simulink library "THAMO_6x2"  (R2018a)
settings: Solver=VariableStepAuto  StartTime=0.0  StopTime=10.0  RelTol=1e-3
undefined symbols (not defined in the file): BM, DiameterLastPiece, DPConstant, DPLinear, DPQuadratic, GeodeticHeight, ID, magnitude, MassFlow, Pressure, Temperature, Water
libraries: carnot x11, simulink x10, $bdroot x3
(part 1 of 3)
settings Model: Creator=volkmer  LastModifiedBy=volkmer
settings CodeAppCC: StateflowObjectComments=on

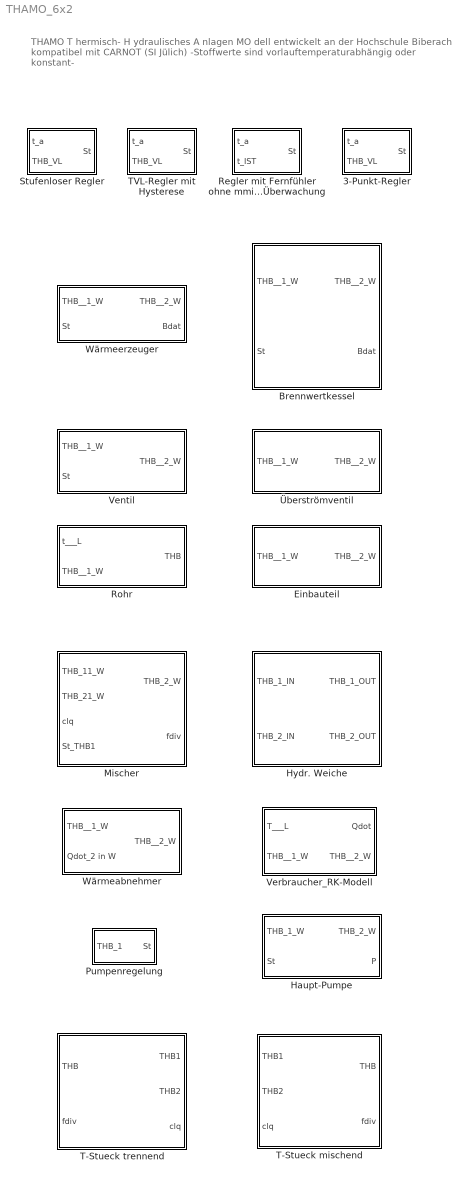
== system THAMO_6x2 ==
  note: THAMO
      | T hermisch- H ydraulisches A nlagen MO dell
      | entwickelt an der Hochschule Biberach
      | kompatibel mit CARNOT (SI Jülich)
      | -Stoffwerte sind vorlauftemperaturabhängig oder konstant-
  3-Punkt-Regler : Subsystem  mask{TVLmax=90, T_HG=50, TVLmin=0, q_S1=40, hyst_S1=6, mmin=3000/30/4.19, tmin=15}
      mask prompts: TVLmax "Vorlauftemperatur bei -16°C"; T_HG "Heizgrenztemperatur"; TVLmin "Vorlauftemperatur bei HG"; q_S1 "Rel. Leistung Stufe 1 in %"; hyst_S1 "Einschaltdifferenz Stufe 1 in K"; mmin "Mindestmassenstrom in kg/s"; tmin "Mindestlaufzeit in min"
      mask DialogControl Container5 Prompt: Heizkurve
      mask DialogControl ParameterGroupVar Prompt: Zusätzliche Parameter
  Brennwertkessel : Subsystem  mask(Condensing Boiler){FUEL=Erdgas, pt_N=20000, V=0.2, Uw=50, AWThw=5, AWTbw=5, P_rel=[20 120], pt_rel=[0.25 1], Lz=1.3, WG_WEhw=4.5, t_hw_A=195, Tamb=20, UV=10, DVB=mit zeta-Wert, kvs=40, zeta=2.5, d=40, m_N=19.44, dp_N=2000}
      mask prompts: FUEL "Brennstoff"; pt_N "Nennleistung in W"; V "Kesselvolumen in m³"; Uw "Wärmedurchgangskoeffizient WÜ in W/m²K"; AWThw "Fläche Kessel-WÜ in m²"; AWTbw "Fläche BW-WÜ in m²"; P_rel "Elektrische Leistung in W (Vektor, index from relative power)"; pt_rel "Rel. Heizleistung in 0..1 (Vektor für P_rel)"; Lz "Luftzahl [-]"; WG_WEhw "Abgasverlust bei t_hw_A in %"; t_hw_A "Abgastemperatur t_hw_A in °C"; Tamb "Umgebungstemperatur in °C"; UV "Wärmeverluste an Umgebung in W/K"; DVB "Druckverlustberechnung"; kvs "kvs-Wert"; zeta "zeta-Wert"; d "Durchmesser in mm"; m_N "Nennmassenstrom in kg/s"; dp_N "Nenndruckverlust in Pa"
      mask help: Multinode one-dimensional model of a boiler. Condensing effects are taken in account by an efficiency lookup table.
      mask Help: web(fullfile(path_carnot('help'),'Condensing_Boiler.html'),'-helpbrowser')
      mask TypeOptions FUEL: Erdgas | Holz (mittel) | Heizoel EL
      mask Callback FUEL:
      | FUEL=1;
      | FUEL=2;
      | FUEL=3;
      mask TypeOptions DVB: mit kvs-Wert | mit zeta-Wert | mit Betriebspunkt
      mask Callback DVB:
      | Auswahl = get_param(gcb,'DVB');
      | Feld = Simulink.Mask.get(gcb);
      | if strcmp(Auswahl,'mit kvs-Wert')
      |     Feld.Parameters(15).Visible = 'on';
      |     Feld.Parameters(16).Visible = 'off';
      |     Feld.Parameters(17).Visible = 'off';
      |     Feld.Parameters(18).Visible = 'off';
      |     Feld.Parameters(19).Visible = 'off';
      |     BM = 1;
      | elseif strcmp(Auswahl,'mit zeta-Wert')
      |     Feld.Parameters(15).Visible = 'off';
      |     Feld.Parameters(16).Visible = 'on';
      |     Feld.Parameters(17).Visible = 'on';
      |     Feld.Parameters(18).Visible = 'off';
      |     Feld.Parameters(19).Visible = 'off';
      |     BM = 2;
      | else
      |     Feld.Parameters(15).Visible = 'off';
      |     Feld.Parameters(16).Visible = 'off';
      |     Feld.Parameters(17).Visible = 'off';
      |     Feld.Parameters(18).Visible = 'on';
      |     Feld.Parameters(19).Visible = 'on';
      |     BM = 3;
      | end
      mask DialogControl DescGroupVar Prompt: Brennwertkessel
      mask DialogControl DescTextVar Prompt: Wärmeerzeuger mit Brennwert-WT für unterschiedliche Brennstoffe
      mask DialogControl ParameterTabVar0 Prompt: Thermisch
      mask DialogControl ParameterTabVar01 Prompt: Effizienz
      mask DialogControl ParameterTabVar012 Prompt: Hydraulisch
      mask Display:
      | plot(-30,0,120,120,[10,90,90,10,10]*0.8,[10,10,20,20,10]*0.8,[80,80,20,20]*0.8,[20,90,90,20]*0.8,[20,70,70,20]*0.8,[24,24,30,30]*0.8,[32,30,28]*0.8,[30,40,30]*0.8,[43,40,38]*0.8,[30,40,30]*0.8,[53,50,47]*0.8,[30,40,30]*0.8,[63,60,57]*0.8,[30,40,30]*0.8,[35,32,30,29,31,36,39,40,37,35]*0.8,[75,69,65,58,50,49,53,59,68,75]*0.8,[57,54,51,51,53,58,62,62,59,57]*0.8,[76,71,67,58,49,48,54,60,69,76]*0.8)
      | port_label('input',1,'THB_1_W')
      | port_label('input',2,'St')
      | port_label('output',1,'THB_2_W')
      | port_label('output',2,'Bdat')
  Einbauteil : Subsystem  mask(Einbauteil){DVB=mit kvs-Wert, kvs=4, zeta=2.5, d=20, m_N=1, dp_N=10^5}
      mask prompts: DVB "Druckverlustberechnung"; kvs "kvs-Wert"; zeta "zeta-Wert"; d "Durchmesser in mm"; m_N "Nennmassenstrom in kg/s"; dp_N "Nenndruckverlust in Pa"
      mask Help: web(fullfile(path_carnot('help'),'Pipe.html'),'-helpbrowser')
      mask TypeOptions DVB: mit kvs-Wert | mit zeta-Wert | mit Betriebspunkt
      mask Callback DVB:
      | Auswahl = get_param(gcb,'DVB');
      | Feld = Simulink.Mask.get(gcb);
      | if strcmp(Auswahl,'mit kvs-Wert')
      |     Feld.Parameters(2).Visible = 'on';
      |     Feld.Parameters(3).Visible = 'off';
      |     Feld.Parameters(4).Visible = 'off';
      |     Feld.Parameters(5).Visible = 'off';
      |     Feld.Parameters(6).Visible = 'off';
      |     BM = 1;
      | elseif strcmp(Auswahl,'mit zeta-Wert')
      |     Feld.Parameters(2).Visible = 'off';
      |     Feld.Parameters(3).Visible = 'on';
      |     Feld.Parameters(4).Visible = 'on';
      |     Feld.Parameters(5).Visible = 'off';
      |     Feld.Parameters(6).Visible = 'off';
      |     BM = 2;
      | else
      |     Feld.Parameters(2).Visible = 'off';
      |     Feld.Parameters(3).Visible = 'off';
      |     Feld.Parameters(4).Visible = 'off';
      |     Feld.Parameters(5).Visible = 'on';
      |     Feld.Parameters(6).Visible = 'on';
      |     BM = 3;
      | end
      mask DialogControl ParameterTabVar0 Prompt: Hydraulik
  Haupt-Pumpe : Subsystem  mask(main pump){a0=651810, a1=5734.30, a2=-346.61, d=0.05, eta_max=80, a=0, mcp=500, p0=4*10^5, IDchk=off, fluid_id=Water, mix=0}
      mask prompts: a0 "Konstanter Kennlinienkoeffizient a0 [Pa]"; a1 "Linearer Kennlinienkoeffizient a1 [Pa*s/kg]"; a2 "Quadratischer Kennlinienkoeffizient a2 [Pa*(s/kg)²]"; d "Anschlussdurchmesser [m]"; eta_max "Max. Wirkungsgrad in %"; a "Wirkungsgradexponent"; mcp "Wärmekapazität in J/K"; p0 "Anlagendruck in Pa"; IDchk "Statischen Druck im System berücksichtigen?"; fluid_id "Fluid"; mix "Mischverhältnis Fluid [0..1]"
      mask help:
      | This is the main pump in a circuit. Every circuit must have exactly ONE 'Pump_Main'. Use the 'pump_additional' blocks if you want to use more pumps.
      | Calculate massflow by solving the equations:
      |     pressure_drop = c + l*mdot + q*(mdot)²
      |     pump_pressure = a0 + a1*mdot +a2*(mdot)²
      |     with: pressure_drop = pump_pressure
      | The system pressure specified as parameter is the pressure at the outlet of the pump. All pressure drops in the circuit will reduce this pressure.
      mask init:
      | ID = IDchk*10000+10001;
      mask Help: web(fullfile(path_carnot('help'),'Pump_Main.html'),'-helpbrowser')
      mask TypeOptions fluid_id: Water | Air | Cotton Oil | Silicone Oil | Water-Glycol Mix | Tyfocor LS | Water (Constant 20°C) | Air (dry+ constant 20°C)
      mask DialogControl ParameterTabVar0 Prompt: Hydraulik
      mask DialogControl Container7 Prompt: Thermisch
      mask DialogControl ParameterTabVar01 Prompt: System
      mask Display:
      | plot(-20,0,100,100,[40,70,40,30,30,40,60,70,70,60,40]*0.8,[70,50,30,40,60,70,70,60,40,30,30]*0.8)
      | 
      | port_label('input',1,'THB_1_W')
      | port_label('input',2,'St')
      | port_label('output',1,'THB_2_W')
      | port_label('output',2,'P')
  Hydr. Weiche : Subsystem  mask{m_HW=500}
      mask prompts: m_HW "Wasserinhalt in kg"
  Mischer : Subsystem  mask{ART=linear, kvs1=4, kvs2=4, dt_V=180}
      mask prompts: ART "Ventilcharakteristik"; kvs1 "kvs THB1-THBg"; kvs2 "kvs THB2-THBg"; dt_V "Mischerlaufzeit in s"
      mask TypeOptions ART: linear | gleichprozentig
      mask Callback ART:
      | ART=1;
      | ART=2;
      mask Display: plot(-25,-5,95,65,[20 45 20 20],[20 30 40 20],[45 70 70 45],[30 20 40 30],[45 35 55 45],[30 10 10 30])
  Pumpenregelung : Subsystem  mask{PUMP=konstantdruckgeregelt, a0=40000, a1=-737, a2=-52000, Vp=20000, Vm=0, nmin=20}
      mask prompts: PUMP "Pumpenbetriebsart"; a0 "constant coefficient in Pa"; a1 "linear coefficient in Pa/(kg/s)"; a2 "quadratic coefficient in Pa/(kg/s)²"; Vp "Vorgabe Förderhöhe (Fußpunkt) in Pa"; Vm "Mindestmassenstrom in kg/s"; nmin "Minimale Drehzahl in %"
      mask TypeOptions PUMP: ungeregelt | konstantdruckgeregelt | proportionaldruckgeregelt
      mask Callback PUMP:
      | PUMP=1;
      | PUMP=2;
      | PUMP=3;
      mask DialogControl DescGroupVar Prompt: Pumpenregelung
      mask DialogControl DescTextVar Prompt: Regelung für eine drehzahlvariable Pumpe
      mask DialogControl ParameterGroupVar Prompt: Reglerdaten
  Regler mit Fernfühler ohne mmin-Überwachung : Subsystem  mask{TVLmax=90, T_HG=50, TVLmin=0, hyst_min=6, tmin=15}
      mask prompts: TVLmax "Vorlauftemperatur bei -16°C"; T_HG "Heizgrenztemperatur"; TVLmin "Vorlauftemperatur bei HG"; hyst_min "Einschaltdifferenz unter Minimalleistung in K"; tmin "Mindestlaufzeit in min"
      mask DialogControl Container5 Prompt: Heizkurve
      mask DialogControl ParameterGroupVar Prompt: Zusätzliche Parameter
  Rohr : Subsystem  mask(Rohr){d=25, L=10, H=0, k=0.03, zeta=0, Uw=20}
      mask prompts: d "Durchmesser in mm"; L "Rohrlänge in m"; H "Wirksame Höhendifferenz in m (offene Systeme)"; k "Rohrrauigkeit in mm"; zeta "zeta-Wert Rohrbögen"; Uw "Wärmeverlust pro m in W/(m*K)"
      mask Help: web(fullfile(path_carnot('help'),'Pipe_Geometry.html'),'-helpbrowser')
      mask DialogControl ParameterTabVar0 Prompt: Hydraulik
      mask DialogControl ParameterTabVar01 Prompt: Thermisch
      mask Display: plot(0,0,90,100,[8,12,16,16,12,8,8],[46,38,46,55,62,55,46],[12,33,48,52,70,73,73,70,50,35,30,12],[38,49,30,30,50,55,65,70,50,70,70,62])
  Stufenloser Regler : Subsystem  mask{TVLmax=90, T_HG=50, TVLmin=0, Kp=50, Ki=6, Kd=3000/30/4.19, q_min=50, hyst_min=6, mmin=3000/30/4.19, tmin=15}
      mask prompts: TVLmax "Vorlauftemperatur bei -16°C"; T_HG "Heizgrenztemperatur"; TVLmin "Vorlauftemperatur bei HG"; Kp "Proportionalbeiwert Kp"; Ki "Integralbeiwert Ki"; Kd "Differentialbeiwert Kd"; q_min "Minimale Leistung in %"; hyst_min "Einschaltdifferenz unter Minimalleistung in K"; mmin "Mindestmassenstrom in kg/s"; tmin "Mindestlaufzeit in min"
      mask DialogControl Container5 Prompt: Heizkurve
      mask DialogControl ParameterGroupVar_copy Prompt: Reglerparameter
      mask DialogControl ParameterGroupVar Prompt: Zusätzliche Parameter
  T-Stueck mischend : Subsystem
      mask Display: plot(-25,-5,95,65,[20 45 20 20],[20 30 40 20],[45 70 70 45],[30 20 40 30],[45 35 55 45],[30 10 10 30])
  T-Stueck trennend : Subsystem  mask(flow diverter, fixed rate){}
      mask help:
      | The block diverts an incoming massflow according to:
      | mdot1 = mdot * fdiv
      | mdot2 = mdot * (1-fdiv)
      | fdiv is limited to the range [0..1]
      mask Help: web(fullfile(path_carnot('help'),'Flow_Diverter.html'),'-helpbrowser')
      mask Display: plot(0,-5,120,65,[20 45 20 20],[20 30 40 20],[45 70 70 45],[30 20 40 30],[45 35 55 45],[30 10 10 30])
  TVL-Regler mit Hysterese : Subsystem  mask{TVLmax=90, T_HG=50, TVLmin=0, hyst_min=6, mmin=3000/30/4.19, tmin=15}
      mask prompts: TVLmax "Vorlauftemperatur bei -16°C"; T_HG "Heizgrenztemperatur"; TVLmin "Vorlauftemperatur bei HG"; hyst_min "Einschaltdifferenz unter Minimalleistung in K"; mmin "Mindestmassenstrom in kg/s"; tmin "Mindestlaufzeit in min"
      mask DialogControl Container5 Prompt: Heizkurve
      mask DialogControl ParameterGroupVar Prompt: Zusätzliche Parameter
  Ventil : Subsystem  mask(Ventil){ART=linear, kvs=5, n_0=0.001, dt_V=180}
      mask prompts: ART "Ventilcharakteristik"; kvs "kvs-Wert in m³/h"; n_0 "Rel. Durchflusskoeffizient"; dt_V "Ventillaufzeit in s"
      mask Help: web(fullfile(path_carnot('help'),'Valve.html'),'-helpbrowser')
      mask TypeOptions ART: linear | gleichprozentig
      mask Callback ART:
      | ART=1;
      | ART=2;
      mask Display: plot(0,10,120,180,[30,70,70,30,30]*0.8,[60,40,60,40,60]*0.8,[60,40]*0.8,[80,80]*0.8,[50,50]*0.8,[50,80]*0.8)
  Verbraucher_RK-Modell : Subsystem  mask(Raumheizeinrichtung){Qdot_N=3*10^6, t_1N=90, t_2N=50, n=1.3, M=500, DVB=mit zeta-Wert, kvs=4, zeta=3, d=150, m_N=1, dp_N=10^5}
      mask prompts: Qdot_N "Nennleistung in W"; t_1N "Nenn-Vorlauftemperatur in °C"; t_2N "Nenn-Rücklauftemperatur in °C"; n "Heizkörperexponent"; M "Wasserinhalt in kg"; DVB "Druckverlustberechnung"; kvs "kvs-Wert"; zeta "zeta-Wert"; d "Durchmesser in mm"; m_N "Nennmassenstrom in kg/s"; dp_N "Nenndruckverlust in Pa"
      mask help: ohne Leistungsvorgabe
      mask Help: web(['file:///' fullfile(path_carnot('help'),'Radiator.html')],'-helpbrowser')
      mask TypeOptions DVB: mit kvs-Wert | mit zeta-Wert | mit Betriebspunkt
      mask Callback DVB:
      | Auswahl = get_param(gcb,'DVB');
      | Feld = Simulink.Mask.get(gcb);
      | if strcmp(Auswahl,'mit kvs-Wert')
      |     Feld.Parameters(7).Visible = 'on';
      |     Feld.Parameters(8).Visible = 'off';
      |     Feld.Parameters(9).Visible = 'off';
      |     Feld.Parameters(10).Visible = 'off';
      |     Feld.Parameters(11).Visible = 'off';
      |     BM = 1;
      | elseif strcmp(Auswahl,'mit zeta-Wert')
      |     Feld.Parameters(7).Visible = 'off';
      |     Feld.Parameters(8).Visible = 'on';
      |     Feld.Parameters(9).Visible = 'on';
      |     Feld.Parameters(10).Visible = 'off';
      |     Feld.Parameters(11).Visible = 'off';
      |     BM = 2;
      | else
      |     Feld.Parameters(7).Visible = 'off';
      |     Feld.Parameters(8).Visible = 'off';
      |     Feld.Parameters(9).Visible = 'off';
      |     Feld.Parameters(10).Visible = 'on';
      |     Feld.Parameters(11).Visible = 'on';
      |     BM = 3;
      | end
      mask DialogControl ParameterTabVar0 Prompt: Thermisch
      mask DialogControl ParameterTabVar01 Prompt: Hydraulik
      mask Display:
      | plot(-20,0,120,90,[20 90 90 20 20],[20 20 70 70 20],[30 30],[25 65],[40 40],[25 65],[50 50],[25 65],[60 60],[25 65],[70 70],[25 65],[80 80],[25 65],[15 20],[25 25],[15 20],[65 65])
      | port_label('input',1,'Troom')
      | port_label('input',2,'THB')
      | port_label('output',1,'Qdot')
      | port_label('output',2,'THB')
  Wärmeabnehmer : Subsystem  mask(Raumheizeinrichtung){M=5, DVB=mit kvs-Wert, kvs=4, zeta=2.5, d=20, m_N=1, dp_N=10^5}
      mask prompts: M "Wasserinhalt in kg"; DVB "Druckverlustberechnung"; kvs "kvs-Wert"; zeta "zeta-Wert"; d "Durchmesser in mm"; m_N "Nennmassenstrom in kg/s"; dp_N "Nenndruckverlust in Pa"
      mask help: mit Leistungsvorgabe (bei Kälte negativ)
      mask Help: web(['file:///' fullfile(path_carnot('help'),'Radiator.html')],'-helpbrowser')
      mask TypeOptions DVB: mit kvs-Wert | mit zeta-Wert | mit Betriebspunkt
      mask Callback DVB:
      | Auswahl = get_param(gcb,'DVB');
      | Feld = Simulink.Mask.get(gcb);
      | if strcmp(Auswahl,'mit kvs-Wert')
      |     Feld.Parameters(3).Visible = 'on';
      |     Feld.Parameters(4).Visible = 'off';
      |     Feld.Parameters(5).Visible = 'off';
      |     Feld.Parameters(6).Visible = 'off';
      |     Feld.Parameters(7).Visible = 'off';
      |     BM = 1;
      | elseif strcmp(Auswahl,'mit zeta-Wert')
      |     Feld.Parameters(3).Visible = 'off';
      |     Feld.Parameters(4).Visible = 'on';
      |     Feld.Parameters(5).Visible = 'on';
      |     Feld.Parameters(6).Visible = 'off';
      |     Feld.Parameters(7).Visible = 'off';
      |     BM = 2;
      | else
      |     Feld.Parameters(3).Visible = 'off';
      |     Feld.Parameters(4).Visible = 'off';
      |     Feld.Parameters(5).Visible = 'off';
      |     Feld.Parameters(6).Visible = 'on';
      |     Feld.Parameters(7).Visible = 'on';
      |     BM = 3;
      | end
      mask DialogControl ParameterTabVar0 Prompt: Thermisch
      mask DialogControl ParameterTabVar01 Prompt: Hydraulik
      mask Display:
      | plot(-20,0,120,90,[20 90 90 20 20],[20 20 70 70 20],[30 30],[25 65],[40 40],[25 65],[50 50],[25 65],[60 60],[25 65],[70 70],[25 65],[80 80],[25 65],[15 20],[25 25],[15 20],[65 65])
      | port_label('input',1,'THB')
      | port_label('input',2,'Qdot_2')
      | port_label('output',1,'THB')
  Wärmeerzeuger : Subsystem  mask(Condensing Boiler){pt_N=20, V=200, FUEL=Erdgas, UV=10, Tamb=20, G=[5 10], t_hw_A=195, WG_WEhw=4.5, Lz=1.3, DVB=mit Betriebspunkt, kvs=40, zeta=2.5, d=40, m_N=1, dp_N=10^5}
      mask prompts: pt_N "Nennleistung in kW"; V "Kesselvolumen in L"; FUEL "Brennstoff"; UV "Wärmeverlust in W/K"; Tamb "Umgebungstemperatur in °C"; G "Grädigkeit Abgas-TRL in K bei Q=[50% 100%]"; t_hw_A "Abgastemperatur t_hw_A in °C"; WG_WEhw "Abgasverlust (ohne Brennwertnutzung) bei Abgastemperatur t_hw_A in %"; Lz "Luftzahl"; DVB "Druckverlustberechnung"; kvs "kvs-Wert"; zeta "zeta-Wert"; d "Durchmesser in mm"; m_N "Nennmassenstrom in kg/s"; dp_N "Nenndruckverlust in Pa"
      mask help: Multinode one-dimensional model of a boiler. Condensing effects are taken in account by an efficiency lookup table.
      mask Help: web(fullfile(path_carnot('help'),'Condensing_Boiler.html'),'-helpbrowser')
      mask TypeOptions FUEL: Erdgas | Holz (mittel) | Heizoel EL
      mask Callback FUEL:
      | FUEL=1;
      | FUEL=2;
      | FUEL=3;
      mask TypeOptions DVB: mit kvs-Wert | mit zeta-Wert | mit Betriebspunkt
      mask Callback DVB:
      | Auswahl = get_param(gcb,'DVB');
      | Feld = Simulink.Mask.get(gcb);
      | if strcmp(Auswahl,'mit kvs-Wert')
      |     Feld.Parameters(11).Visible = 'on';
      |     Feld.Parameters(12).Visible = 'off';
      |     Feld.Parameters(13).Visible = 'off';
      |     Feld.Parameters(14).Visible = 'off';
      |     Feld.Parameters(15).Visible = 'off';
      |     BM = 1;
      | elseif strcmp(Auswahl,'mit zeta-Wert')
      |     Feld.Parameters(11).Visible = 'off';
      |     Feld.Parameters(12).Visible = 'on';
      |     Feld.Parameters(13).Visible = 'on';
      |     Feld.Parameters(14).Visible = 'off';
      |     Feld.Parameters(15).Visible = 'off';
      |     BM = 2;
      | else
      |     Feld.Parameters(11).Visible = 'off';
      |     Feld.Parameters(12).Visible = 'off';
      |     Feld.Parameters(13).Visible = 'off';
      |     Feld.Parameters(14).Visible = 'on';
      |     Feld.Parameters(15).Visible = 'on';
      |     BM = 3;
      | end
      mask DialogControl DescGroupVar Prompt: Brennwertkessel
      mask DialogControl DescTextVar Prompt: Wärmeerzeuger mit Brennwert-WT für unterschiedliche Brennstoffe
      mask DialogControl ParameterTabVar0 Prompt: Thermisch
      mask DialogControl Container10 Prompt: Effizienz
      mask DialogControl ParameterTabVar012 Prompt: Hydraulisch
  Überströmventil : Subsystem  mask(Überströmventil){p0=27111, p1=1330, p2=1889}
      mask prompts: p0 "Durchbrechdruck in Pa"; p1 "Linearer Druckverlustkoeffizient in Pa/(kg/s)"; p2 "Quadratischer Druckverlustkoeffizient in Pa/(kg/s)^2"
      mask Help: web(fullfile(path_carnot('help'),'Valve.html'),'-helpbrowser')

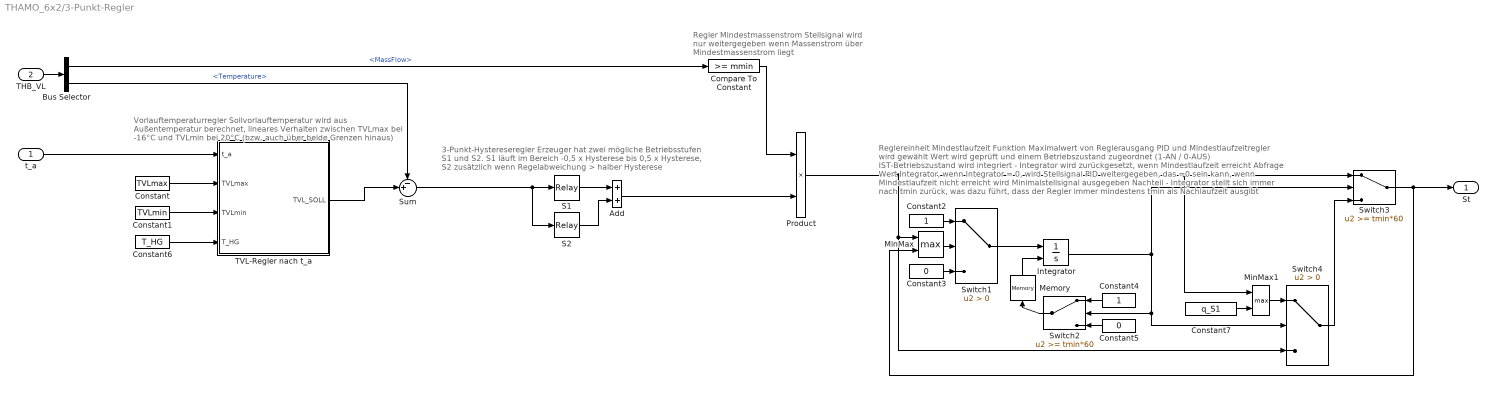
== system THAMO_6x2/3-Punkt-Regler ==
  note: 3-Punkt-Hystereseregler
      |
      | Erzeuger hat zwei mögliche Betriebsstufen
      | S1 und S2. S1 läuft im Bereich -0,5 x Hysterese bis 0,5 x Hysterese, S2 zusätzlich wenn Regelabweichung > halber Hysterese
  note: Vorlauftemperaturregler
      |
      | Sollvorlauftemperatur wird aus Außentemperatur berechnet, lineares Verhalten zwischen TVLmax bei -16°C und TVLmin bei 20°C (bzw. auch über beide Grenzen hinaus)
  note: Regler Mindestmassenstrom
      |
      | Stellsignal wird nur weitergegeben wenn Massenstrom über Mindestmassenstrom liegt
  note: Reglereinheit Mindestlaufzeit
      |
      | Funktion
      | Maximalwert von Reglerausgang PID und Mindestlaufzeitregler wird gewählt
      | Wert wird geprüft und einem Betriebszustand zugeordnet (1-AN / 0-AUS)
      | IST-Betriebszustand wird integriert - Integrator wird zurückgesetzt, wenn Mindestlaufzeit erreicht
      | Abfrage Wert Integrator, wenn Integrator = 0, wird Stellsignal PID weitergegeben, das =0 sein kann, wenn Mindestlaufzeit nicht erreicht wird Minimalstellsignal ausgegeben
      |
      | Nachteil
      | - Integrator stellt sich immer nach tmin zurück, was dazu führt, dass der Regler immer mindestens tmin als Nachlaufzeit ausgibt
  t_a : Inport
  THB_VL : Inport  Port=2
  Add : Sum
  Bus Selector : BusSelector  OutputSignals=MassFlow,Temperature
  Compare To Constant : simulink/Logic and Bit Operations/Compare To Constant  relop=>=  const=mmin  OutDataTypeStr=boolean
  Constant : Constant  Value=TVLmax
  Constant1 : Constant  Value=TVLmin
  Constant2 : Constant
  Constant3 : Constant  Value=0
  Constant4 : Constant
  Constant5 : Constant  Value=0
  Constant6 : Constant  Value=T_HG
  Constant7 : Constant  Value=q_S1
  Integrator : Integrator  ExternalReset=level hold
  Memory : Memory  InitialCondition=1
  MinMax : MinMax  Function=max  Inputs=2
  MinMax1 : MinMax  Function=max  Inputs=2
  Product : Product
  S1 : Relay  OnSwitchValue=hyst_S1*0.5  OffSwitchValue=-hyst_S1*0.5  OnOutputValue=q_S1/100
  S2 : Relay  OnSwitchValue=hyst_S1  OffSwitchValue=-hyst_S1*0.5  OnOutputValue=1-q_S1/100
  Sum : Sum  Inputs=-+|
  Switch1 : Switch  Criteria=u2 > Threshold
  Switch2 : Switch  Threshold=tmin*60
  Switch3 : Switch  Threshold=tmin*60
  Switch4 : Switch  Criteria=u2 > Threshold
  TVL-Regler nach t_a : MATLAB Function  TreatAsAtomicUnit=on
  St : Outport
  wires:
  Memory/1 -> Integrator/2
  TVL-Regler nach t_a/1(TVL_SOLL) -> Sum/2
  Compare To Constant/1 -> Product/1
  Bus Selector/1 -> Compare To Constant/1  "<MassFlow>"
  Product/1 -> MinMax1/1, Switch3/1, Switch4/3, MinMax/1
  Constant1/1 -> TVL-Regler nach t_a/3(TVLmin)
  Constant/1 -> TVL-Regler nach t_a/2(TVLmax)
  t_a/1 -> TVL-Regler nach t_a/1(t_a)
  Bus Selector/2 -> Sum/1  "<Temperature>"
  THB_VL/1 -> Bus Selector/1
  Constant2/1 -> Switch1/1
  Constant3/1 -> Switch1/3
  Switch1/1 -> Integrator/1
  Switch2/1 -> Memory/1
  Constant4/1 -> Switch2/1
  Constant5/1 -> Switch2/3
  Integrator/1 -> Switch2/2, Switch4/2, Switch3/2
  Switch3/1 -> St/1, MinMax/2
  Switch4/1 -> Switch3/3
  MinMax/1 -> Switch1/2
  MinMax1/1 -> Switch4/1
  Constant7/1 -> MinMax1/2
  Add/1 -> Product/2
  S2/1 -> Add/2
  Sum/1 -> S1/1, S2/1
  S1/1 -> Add/1
  Constant6/1 -> TVL-Regler nach t_a/4(T_HG)

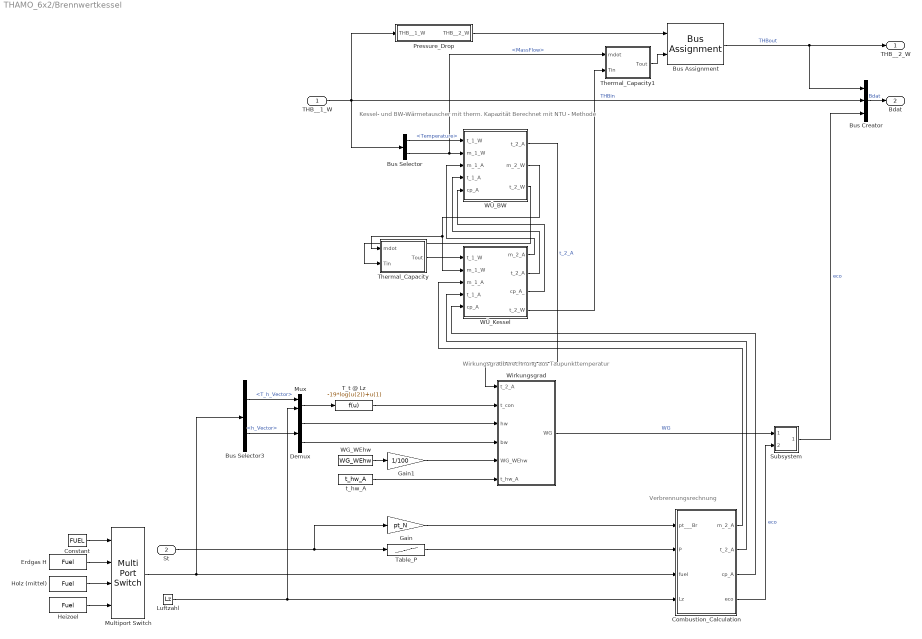
== system THAMO_6x2/Brennwertkessel ==
  note: Wirkungsgradberechnung aus Taupunkttemperatur
  note: Verbrennungsrechnung
  note: Kessel- und BW-Wärmetauscher mit therm. Kapazität
      |
      | Berechnet mit NTU - Methode
  THB__1_W : Inport
  St : Inport  Port=2
  Bus Assignment : BusAssignment  AssignedSignals=Temperature
  Bus Creator : BusCreator  Inputs=3
  Bus Selector : BusSelector  OutputSignals=Temperature,MassFlow
  Bus Selector3 : BusSelector  OutputSignals=T_h_Vector,h_Vector
  Combustion_Calculation : Subsystem  TreatAsAtomicUnit=on
  Constant : Constant  Value=FUEL
  Demux : Demux  Outputs=2
  Erdgas H : carnot/Source/Energy/Fuel  ft=1  t=20  ls=15.59  p=1e5  h_values=[38.5 43]*10^6  tc=57.53  price=1  mass=[0.22 0.70 0.05 0 0.03 0]
  Gain : Gain  Gain=pt_N
  Gain1 : Gain  Gain=1/100
  Heizoel : carnot/Source/Energy/Fuel  ft=2  t=20  ls=15.94  p=1e5  h_values=[42.6 45.4]*10^6  tc=50.37  price=1  mass=[0.13 0.87 0 0 0 0]
  Holz (mittel) : carnot/Source/Energy/Fuel  ft=3  t=20  ls=6.54  p=1e5  h_values=[15.1 19]*10^6  tc=67.5  price=1  mass=[0.06 0.5 0.44 0 0 0]
  Luftzahl : Constant  Value=Lz
  Multiport Switch : MultiPortSwitch
  Mux : Mux  Inputs=2
  Pressure_Drop : Subsystem  mask(fixed pressure drop){}
      mask help:
      | Constant parameters for pressure drop in a flow.
      | dp = c + l*mdot + q*mdot²
      | Calculation is done for ID > 10000 (dp = f(l, q), c is neglected) and ID > 20000 (dp = f(c,l,q)).
      | Applied directly to the THB bus.
      mask Help: web(fullfile(path_carnot('help'),'Pressure_Drop_Fix.html'),'-helpbrowser')
  Subsystem : Subsystem
  T_t @ Lz : Fcn  Expr=-19*log(u(2))+u(1)
  Table_P : Lookup_n-D  NumberOfTableDimensions=1  BreakpointsForDimension1=[0 pt_rel]  Table=[0 P_rel]  InternalRulePriority=Speed  InputSameDT=on
  Thermal_Capacity : Subsystem  mask(Thermal Capacity){}
      mask help: Basic one node model of a thermal mass using the differential equation:
      mask Help: web(fullfile(path_carnot('help'),'Thermal_Capacity.html'),'-helpbrowser')
  Thermal_Capacity1 : Subsystem  mask(Thermal Capacity){}
      mask help: Basic one node model of a thermal mass using the differential equation:
      mask Help: web(fullfile(path_carnot('help'),'Thermal_Capacity.html'),'-helpbrowser')
  WG_WEhw : Constant  Value=WG_WEhw
  Wirkungsgrad : MATLAB Function  TreatAsAtomicUnit=on
  WÜ_BW : Subsystem
  WÜ_Kessel : Subsystem
  t_hw_A : Constant  Value=t_hw_A
  THB__2_W : Outport
  Bdat : Outport  Port=2
  wires:
  Combustion_Calculation/2(t_2_A) -> WÜ_Kessel/4(t_1_A)
  Constant/1 -> Multiport Switch/1
  Heizoel/1 -> Multiport Switch/4
  Holz (mittel)/1 -> Multiport Switch/3
  Erdgas H/1 -> Multiport Switch/2
  Combustion_Calculation/1(m_2_A) -> WÜ_Kessel/3(m_1_A)
  WÜ_BW/1(t_2_A) -> Wirkungsgrad/1(t_2_A)  "t_2_A"
  Gain1/1 -> Wirkungsgrad/5(WG_WEhw)
  t_hw_A/1 -> Wirkungsgrad/6(t_hw_A)
  WG_WEhw/1 -> Gain1/1
  T_t @ Lz/1 -> Wirkungsgrad/2(t_con)
  Luftzahl/1 -> Mux/2, Combustion_Calculation/4(Lz)
  Mux/1 -> T_t @ Lz/1
  Demux/2 -> Wirkungsgrad/4(bw)
  Demux/1 -> Wirkungsgrad/3(hw)
  Bus Selector3/2 -> Demux/1  "<h_Vector>"
  Bus Selector3/1 -> Mux/1  "<T_h_Vector>"
  Table_P/1 -> Combustion_Calculation/2(P)
  Bus Creator/1 -> Bdat/1  "Bdat"
  THB__1_W/1 -> Bus Selector/1, Pressure_Drop/1(THB__1_W), Bus Creator/2  "THBin"
  Bus Assignment/1 -> THB__2_W/1, Bus Creator/1  "THBout"
  St/1 -> Table_P/1, Gain/1
  Multiport Switch/1 -> Bus Selector3/1, Combustion_Calculation/3(fuel)
  Pressure_Drop/1(THB__2_W) -> Bus Assignment/1
  Gain/1 -> Combustion_Calculation/1(pt___Br)
  Bus Selector/2 -> Thermal_Capacity1/1(mdot), WÜ_BW/2(m_1_W)  "<MassFlow>"
  WÜ_BW/2(m_2_W) -> WÜ_Kessel/2(m_1_W), Thermal_Capacity/1(mdot)
  Combustion_Calculation/3(cp_A) -> WÜ_Kessel/5(cp_A)
  WÜ_Kessel/3(cp_A_) -> WÜ_BW/5(cp_A)
  Wirkungsgrad/1(WG) -> Subsystem/1(WG)  "WG"
  Combustion_Calculation/4(eco) -> Subsystem/2(eco_in)  "eco"
  Subsystem/1(eco) -> Bus Creator/3  "eco"
  WÜ_Kessel/1(m_2_A) -> WÜ_BW/3(m_1_A)
  Bus Selector/1 -> WÜ_BW/1(t_1_W)  "<Temperature>"
  WÜ_Kessel/2(t_2_A) -> WÜ_BW/4(t_1_A)
  WÜ_BW/3(t_2_W) -> Thermal_Capacity/2(Tin)
  WÜ_Kessel/4(t_2_W) -> Thermal_Capacity1/2(Tin)
  Thermal_Capacity/1(Tout) -> WÜ_Kessel/1(t_1_W)
  Thermal_Capacity1/1(Tout) -> Bus Assignment/2

== system THAMO_6x2/Einbauteil ==
  THB__1_W : Inport
  Pressure_Drop : $bdroot/Brennwertkessel/Pressure_Drop
  THB__2_W : Outport
  wires:
  Pressure_Drop/1 -> THB__2_W/1
  THB__1_W/1 -> Pressure_Drop/1

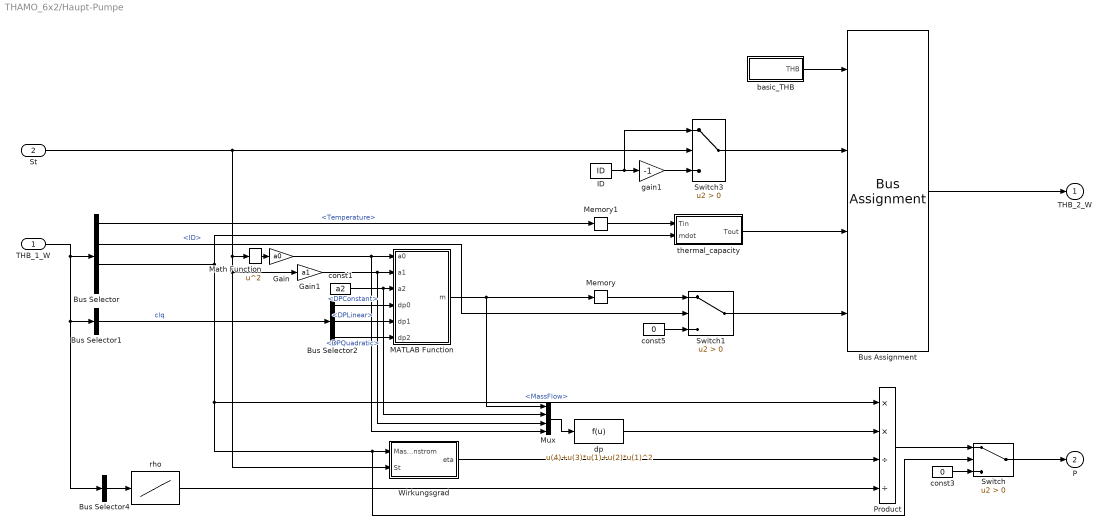
== system THAMO_6x2/Haupt-Pumpe ==
  THB_1_W : Inport
  St : Inport  Port=2
  Bus Assignment : BusAssignment  AssignedSignals=ID,Temperature,MassFlow
  Bus Selector : BusSelector  OutputSignals=Temperature,ID,MassFlow,Pressure
  Bus Selector1 : BusSelector  OutputSignals=DPQuadratic,DPLinear,DPConstant  OutputAsBus=on
  Bus Selector2 : BusSelector  OutputSignals=DPConstant,DPLinear,DPQuadratic
  Bus Selector4 : BusSelector  OutputSignals=Temperature  OutputAsBus=on
  Gain : Gain  Gain=a0
  Gain1 : Gain  Gain=a1
  ID : Constant  Value=ID
  MATLAB Function : MATLAB Function  TreatAsAtomicUnit=on
  Math Function : Math  Operator=square  SaturateOnIntegerOverflow=on
  Memory : Memory  InitialCondition=10^-9
  Memory1 : Memory  InitialCondition=20
  Mux : Mux
  Product : Product  Inputs=**//  SaturateOnIntegerOverflow=on  InputSameDT=on  OutDataTypeStr=Inherit: Same as first input
  Switch : Switch  Criteria=u2 > Threshold
  Switch1 : Switch  Criteria=u2 > Threshold  SaturateOnIntegerOverflow=on  InputSameDT=on
  Switch3 : Switch  Criteria=u2 > Threshold  SaturateOnIntegerOverflow=on  InputSameDT=on
  Wirkungsgrad : Subsystem
  basic_THB : Subsystem  mask(basic THB){t=20, mdot=0, p=p0, ID=Pressure Drop from Massflow, fluid=Water, mix=mix, mix2=0, mix3=0, dia=d, hgt=0}
      mask prompts: t "temperature [°C]"; mdot "massflow [kg/s]"; p "pressure [Pa]"; ID "ID for pressure drop calculation"; mix "fluid mixture [0..1]"; mix2 "fluid mixture 2 [0..1]"; mix3 "fluid mixture 3 [0..1]"; dia "diameter [m]"; hgt "Static height in m"
      mask help:
      | Create a constant Thermo-Hydraulic-Vector.
      | Pressure drop calculation mode (defined by ID):
      |     1 ..  9999 no pressure drop (dp)
      | 10001 .. 19999 dp caused by flowrate
      | 20001 .. inf   dp by flowrate and static height
      mask Help: web(fullfile(path_carnot('help'),'basic_THB.html'),'-helpbrowser')
      mask TypeOptions t: const24/Value
      mask TypeOptions mdot: const25/Value
      mask TypeOptions p: const26/Value
      mask TypeOptions ID: const21/mID
      mask TypeOptions fluid: const27/fluid
      mask TypeOptions mix: const28/Value
      mask TypeOptions mix2: const2/Value
      mask TypeOptions mix3: const3/Value
      mask TypeOptions dia: const29/Value
      mask TypeOptions hgt: const1/Value
      mask DialogControl ParameterTabVar0 Prompt: Hydraulic
      mask DialogControl ParameterTabVar01 Prompt: Fluid
      mask DialogControl ParameterTabVar012 Prompt: Geometry
  const1 : Constant  Value=a2
  const3 : Constant  Value=0
  const5 : Constant  Value=0
  dp : Fcn  Expr=u(4)+u(3)*u(1)+u(2)*u(1)^2
  gain1 : Gain  Gain=-1  SaturateOnIntegerOverflow=on  OutDataTypeStr=Inherit: Same as input  ParamDataTypeStr=Inherit: Same as input
  rho : Lookup_n-D  NumberOfTableDimensions=1  BreakpointsForDimension1=[0,10,20,30,40,50,60,70,80,90,100]  Table=[999.84,999.7,998.2,995.64,992.21,988.03,983.19,977.76,971.79,965.3,958.35]  InternalRulePriority=Speed  RndMeth=Simplest  InputSameDT=on
  thermal_capacity : Subsystem  mask(Thermal Capacity){}
      mask help: Basic one node model of a thermal mass using the differential equation:
      mask Help: web(fullfile(path_carnot('help'),'Thermal_Capacity.html'),'-helpbrowser')
  THB_2_W : Outport
  P : Outport  Port=2
  wires:
  Bus Selector4/1 -> rho/1
  Memory1/1 -> thermal_capacity/1(Tin)
  Gain/1 -> Mux/4, MATLAB Function/1(a0)
  const1/1 -> Mux/2, MATLAB Function/3(a2)
  Bus Selector2/3 -> MATLAB Function/6(dp2)  "<DPQuadratic>"
  Bus Selector2/2 -> MATLAB Function/5(dp1)  "<DPLinear>"
  Bus Selector2/1 -> MATLAB Function/4(dp0)  "<DPConstant>"
  MATLAB Function/1(m) -> Mux/1, Memory/1
  Memory/1 -> Switch1/1
  Gain1/1 -> Mux/3, MATLAB Function/2(a1)
  Math Function/1 -> Gain/1
  Wirkungsgrad/1(eta) -> Product/3
  rho/1 -> Product/4
  Bus Selector/3 -> thermal_capacity/2(mdot), Wirkungsgrad/1(Massenstrom), Switch/2, Product/1  "<MassFlow>"
  Bus Selector1/1 -> Bus Selector2/1  "clq"
  THB_1_W/1 -> Bus Selector4/1, Bus Selector1/1, Bus Selector/1
  Switch1/1 -> Bus Assignment/4
  Switch3/1 -> Bus Assignment/2
  Bus Assignment/1 -> THB_2_W/1
  basic_THB/1(THB) -> Bus Assignment/1
  const5/1 -> Switch1/3
  gain1/1 -> Switch3/3
  ID/1 -> gain1/1, Switch3/1
  St/1 -> Switch3/2, Wirkungsgrad/2(St), Gain1/1, Math Function/1
  Bus Selector/2 -> Switch1/2  "<ID>"
  Product/1 -> Switch/1
  thermal_capacity/1(Tout) -> Bus Assignment/3
  Bus Selector/1 -> Memory1/1  "<Temperature>"
  Switch/1 -> P/1
  const3/1 -> Switch/3
  Mux/1 -> dp/1
  dp/1 -> Product/2

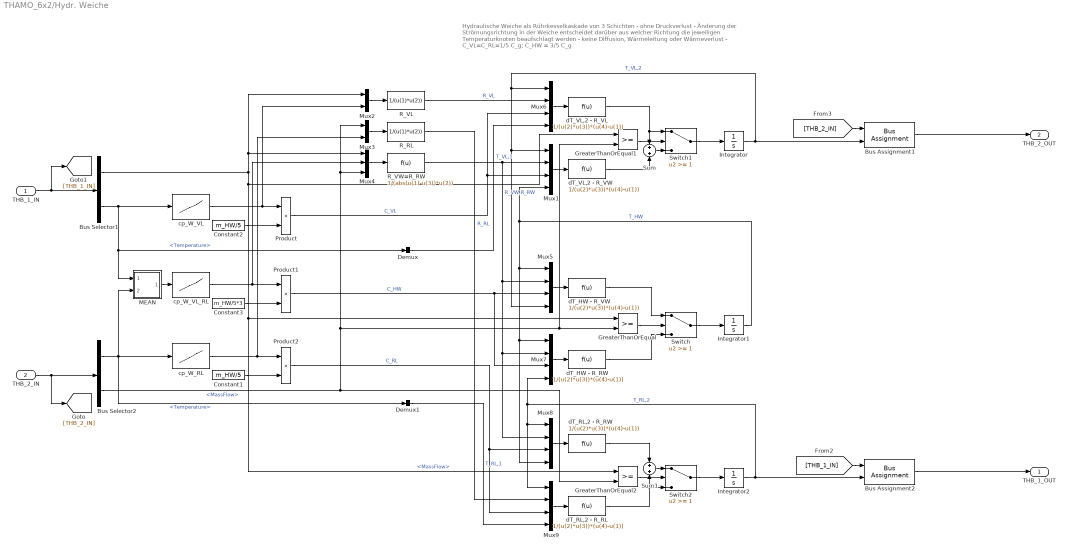
== system THAMO_6x2/Hydr. Weiche ==
  note: Hydraulische Weiche als Rührkesselkaskade von 3 Schichten
      | - ohne Druckverlust
      | - Änderung der Strömungsrichtung in der Weiche entscheidet darüber aus welcher Richtung die jeweiligen Temperaturknoten beaufschlagt werden
      | - keine Diffusion, Wärmeleitung oder Wärmeverlust
      | - C_VL=C_RL=1/5 C_g; C_HW = 3/5 C_g
  THB_1_IN : Inport
  THB_2_IN : Inport  Port=2
  Bus Assignment1 : BusAssignment  AssignedSignals=Temperature
  Bus Assignment2 : BusAssignment  AssignedSignals=Temperature
  Bus Selector1 : BusSelector  OutputSignals=MassFlow,Temperature
  Bus Selector2 : BusSelector  OutputSignals=Temperature,MassFlow
  Constant1 : Constant  Value=m_HW/5
  Constant2 : Constant  Value=m_HW/5
  Constant3 : Constant  Value=m_HW/5*3
  Demux : Demux  Outputs=1
  Demux1 : Demux  Outputs=1
  GreaterThanOrEqual : RelationalOperator  OutDataTypeStr=boolean  RndMeth=Simplest
  GreaterThanOrEqual1 : RelationalOperator  OutDataTypeStr=boolean  RndMeth=Simplest
  GreaterThanOrEqual2 : RelationalOperator  OutDataTypeStr=boolean  RndMeth=Simplest
  Integrator : Integrator  InitialCondition=20
  Integrator1 : Integrator  InitialCondition=20
  Integrator2 : Integrator  InitialCondition=20
  MEAN : Subsystem
  Mux{1,5..9} (6 alike) : Mux
  Mux2 : Mux  Inputs=2
  Mux3 : Mux  Inputs=2
  Mux4 : Mux  Inputs=3
  Product : Product
  Product1 : Product
  Product2 : Product
  R_RL : Fcn  Expr=1/(u(1)*u(2))
  R_VL : Fcn  Expr=1/(u(1)*u(2))
  R_VW=R_RW : Fcn  Expr=1/(abs(u(1)-u(3))*u(2))
  Sum : Sum  Inputs=+|+
  Sum1 : Sum  Inputs=+|+
  Switch : Switch  Threshold=1
  Switch1 : Switch  Threshold=1
  Switch2 : Switch  Threshold=1
  cp_W_RL : Lookup_n-D  NumberOfTableDimensions=1  BreakpointsForDimension1=[0,10,20,30,40,50,60,70,80,90,100]  Table=[4218,4192,4182,4179,4179,4181,4184,4190,4196,4205,4216]  InternalRulePriority=Speed  RndMeth=Simplest  InputSameDT=on
  cp_W_VL : Lookup_n-D  NumberOfTableDimensions=1  BreakpointsForDimension1=[0,10,20,30,40,50,60,70,80,90,100]  Table=[4218,4192,4182,4179,4179,4181,4184,4190,4196,4205,4216]  InternalRulePriority=Speed  RndMeth=Simplest  InputSameDT=on
  cp_W_VL_RL : Lookup_n-D  NumberOfTableDimensions=1  BreakpointsForDimension1=[0,10,20,30,40,50,60,70,80,90,100]  Table=[4218,4192,4182,4179,4179,4181,4184,4190,4196,4205,4216]  InternalRulePriority=Speed  RndMeth=Simplest  InputSameDT=on
  dT_HW - R_RW : Fcn  Expr=1/(u(2)*u(3))*(u(4)-u(1))
  dT_HW - R_VW : Fcn  Expr=1/(u(2)*u(3))*(u(4)-u(1))
  dT_RL,2 - R_RL : Fcn  Expr=1/(u(2)*u(3))*(u(4)-u(1))
  dT_RL,2 - R_RW : Fcn  Expr=1/(u(2)*u(3))*(u(4)-u(1))
  dT_VL,2 - R_VL : Fcn  Expr=1/(u(2)*u(3))*(u(4)-u(1))
  dT_VL,2 - R_VW : Fcn  Expr=1/(u(2)*u(3))*(u(4)-u(1))
  THB_1_OUT : Outport
  THB_2_OUT : Outport  Port=2
  wires:
  Bus Assignment2/1 -> THB_1_OUT/1
  Bus Assignment1/1 -> THB_2_OUT/1
  dT_HW - R_RW/1 -> Switch/3
  dT_HW - R_VW/1 -> Switch/1
  dT_RL,2 - R_RL/1 -> Sum1/2, Switch2/3
  dT_RL,2 - R_RW/1 -> Sum1/1
  Sum1/1 -> Switch2/1
  dT_VL,2 - R_VW/1 -> Sum/2
  dT_VL,2 - R_VL/1 -> Sum/1, Switch1/1
  Sum/1 -> Switch1/3
  Switch2/1 -> Integrator2/1
  Switch1/1 -> Integrator/1
  GreaterThanOrEqual2/1 -> Switch2/2
  GreaterThanOrEqual1/1 -> Switch1/2
  Switch/1 -> Integrator1/1
  GreaterThanOrEqual/1 -> Switch/2
  R_RL/1 -> Mux9/2  "R_RL"
  Integrator2/1 -> Mux7/4, Mux9/1, Mux8/1, Bus Assignment2/2  "T_RL,2"
  Integrator1/1 -> Mux1/4, Mux8/4, Mux7/1, Mux5/1  "T_HW"
  Integrator/1 -> Mux1/1, Mux5/4, Mux6/1, Bus Assignment1/2  "T_VL,2"
  R_VW=R_RW/1 -> Mux1/2, Mux8/2, Mux7/2, Mux5/2  "R_VW,R_RW"
  R_VL/1 -> Mux6/2  "R_VL"
  Mux9/1 -> dT_RL,2 - R_RL/1
  Mux8/1 -> dT_RL,2 - R_RW/1
  Mux7/1 -> dT_HW - R_RW/1
  Mux5/1 -> dT_HW - R_VW/1
  Mux1/1 -> dT_VL,2 - R_VW/1
  Mux6/1 -> dT_VL,2 - R_VL/1
  Product2/1 -> Mux9/3, Mux8/3  "C_RL"
  Product/1 -> Mux1/3, Mux6/3  "C_VL"
  Product1/1 -> Mux5/3, Mux7/3  "C_HW"
  Demux/1 -> Mux6/4  "T_VL,1"
  Demux1/1 -> Mux9/4  "T_RL,1"
  Bus Selector1/1 -> Mux4/1, Mux2/1, GreaterThanOrEqual1/1, GreaterThanOrEqual/1, GreaterThanOrEqual2/1  "<MassFlow>"
  Bus Selector2/2 -> Mux4/3, Mux3/1, GreaterThanOrEqual/2, GreaterThanOrEqual1/2, GreaterThanOrEqual2/2  "<MassFlow>"
  Mux4/1 -> R_VW=R_RW/1
  Mux3/1 -> R_RL/1
  Mux2/1 -> R_VL/1
  [THB_2_IN] -> Bus Assignment1/1
  [THB_1_IN] -> Bus Assignment2/1
  cp_W_RL/1 -> Mux3/2, Product2/1
  Constant1/1 -> Product2/2
  cp_W_VL_RL/1 -> Mux4/2, Product1/1
  Constant3/1 -> Product1/2
  cp_W_VL/1 -> Mux2/2, Product/1
  Constant2/1 -> Product/2
  MEAN/1(Tm) -> cp_W_VL_RL/1
  Bus Selector2/1 -> cp_W_RL/1, Demux1/1, MEAN/2(T_RL)  "<Temperature>"
  Bus Selector1/2 -> cp_W_VL/1, Demux/1, MEAN/1(T_VL)  "<Temperature>"
  THB_1_IN/1 -> Bus Selector1/1, [THB_1_IN]
  THB_2_IN/1 -> Bus Selector2/1, [THB_2_IN]

== system THAMO_6x2/Mischer ==
  note: Zwei Ventile mit möglicherweise unterschiedlichen kvs-Werten (aber gleicher Charakteristik und Laufzeit), wobei St für die Strömung THB_11_W angesetzt wird und das Ventil in THB_21_W entsprechend gegenläufig arbeitet
  THB_11_W : Inport
  THB_21_W : Inport  Port=2
  clq : Inport  Port=3
  St_THB1 : Inport  Port=4
  Constant : Constant
  Sum : Sum  Inputs=-+|
  T-Stueck mischend : $bdroot/T-Stueck mischend  SystemSampleTime=-1
  Ventil : Subsystem  mask(Ventil){kvs=kvs1, n_0=0.01, dt_V=dt_V}
      mask prompts: kvs "kvs-Wert in m³/h"; n_0 "Rel. Durchflusskoeffizient"; dt_V "Ventillaufzeit in s"
      mask Help: web(fullfile(path_carnot('help'),'Valve.html'),'-helpbrowser')
      mask Display: plot(0,10,120,180,[30,70,70,30,30]*0.8,[60,40,60,40,60]*0.8,[60,40]*0.8,[80,80]*0.8,[50,50]*0.8,[50,80]*0.8)
  Ventil1 : Subsystem  mask(Ventil){kvs=kvs2, n_0=0.01, dt_V=dt_V}
      mask prompts: kvs "kvs-Wert in m³/h"; n_0 "Rel. Durchflusskoeffizient"; dt_V "Ventillaufzeit in s"
      mask Help: web(fullfile(path_carnot('help'),'Valve.html'),'-helpbrowser')
      mask Display: plot(0,10,120,180,[30,70,70,30,30]*0.8,[60,40,60,40,60]*0.8,[60,40]*0.8,[80,80]*0.8,[50,50]*0.8,[50,80]*0.8)
  THB_2_W : Outport
  fdiv : Outport  Port=2
  wires:
  THB_21_W/1 -> Ventil1/1(THB__1_W)
  Ventil/1(THB__2_W) -> T-Stueck mischend/1
  Ventil1/1(THB__2_W) -> T-Stueck mischend/2
  THB_11_W/1 -> Ventil/1(THB__1_W)
  T-Stueck mischend/2 -> fdiv/1
  T-Stueck mischend/1 -> THB_2_W/1
  St_THB1/1 -> Sum/1, Ventil/2(St)
  clq/1 -> T-Stueck mischend/3
  Sum/1 -> Ventil1/2(St)
  Constant/1 -> Sum/2

== system THAMO_6x2/Pumpenregelung ==
  THB_1 : Inport
  Bus Selector : BusSelector  OutputSignals=DPConstant,DPLinear,DPQuadratic
  Constant : Constant  Value=a0
  Constant1 : Constant  Value=a1
  Constant2 : Constant  Value=a2
  Constant3 : Constant  Value=Vp
  Constant4 : Constant  Value=Vm
  Constant5 : Constant  Value=PUMP
  Constant6 : Constant  Value=0
  MATLAB Function : MATLAB Function  TreatAsAtomicUnit=on
  Memory : Memory  InitialCondition=1
  Saturation : Saturate  UpperLimit=1  LowerLimit=0  LinearizeAsGain=off
  Switch : Switch  Criteria=u2 > Threshold  Threshold=nmin/100
  St : Outport
  wires:
  MATLAB Function/1(St) -> Switch/1, Switch/2
  Switch/1 -> Saturation/1
  THB_1/1 -> Bus Selector/1
  Bus Selector/1 -> MATLAB Function/1(dp0)  "<DPConstant>"
  Bus Selector/2 -> MATLAB Function/2(dp1)  "<DPLinear>"
  Bus Selector/3 -> MATLAB Function/3(dp2)  "<DPQuadratic>"
  Constant5/1 -> MATLAB Function/4(PUMP)
  Constant/1 -> MATLAB Function/5(a0)
  Constant1/1 -> MATLAB Function/6(a1)
  Constant2/1 -> MATLAB Function/7(a2)
  Constant3/1 -> MATLAB Function/8(Vp)
  Constant4/1 -> MATLAB Function/9(Vm)
  Saturation/1 -> Memory/1
  Memory/1 -> St/1
  Constant6/1 -> Switch/3

== system THAMO_6x2/Regler mit Fernfühler ohne mmin-Überwachung ==
  note: Hystereseregler
      |
      | Erzeuger wird zwischen 0 und 1 mit Hysterese stufig geschalten
  note: Vorlauftemperaturregler
      |
      | Sollvorlauftemperatur wird aus Außentemperatur berechnet, lineares Verhalten zwischen TVLmax bei -16°C und TVLmin bei 20°C (bzw. auch über beide Grenzen hinaus)
  note: Reglereinheit Mindestlaufzeit
      |
      | Funktion
      | Maximalwert von Reglerausgang PID und Mindestlaufzeitregler wird gewählt
      | Wert wird geprüft und einem Betriebszustand zugeordnet (1-AN / 0-AUS)
      | IST-Betriebszustand wird integriert - Integrator wird zurückgesetzt, wenn Mindestlaufzeit erreicht
      | Abfrage Wert Integrator, wenn Integrator = 0, wird Stellsignal PID weitergegeben, das =0 sein kann, wenn Mindestlaufzeit nicht erreicht wird Minimalstellsignal ausgegeben
      |
      | Nachteil
      | - Integrator stellt sich immer nach tmin zurück, was dazu führt, dass der Regler immer mindestens tmin als Nachlaufzeit ausgibt
  t_a : Inport
  t_IST : Inport  Port=2
  Constant : Constant  Value=TVLmax
  Constant1 : Constant  Value=TVLmin
  Constant2 : Constant
  Constant3 : Constant  Value=0
  Constant4 : Constant
  Constant5 : Constant  Value=0
  Constant6 : Constant  Value=T_HG
  Constant7 : Constant
  Integrator : Integrator  ExternalReset=level hold
  Memory : Memory  InitialCondition=1
  MinMax : MinMax  Function=max  Inputs=2
  MinMax1 : MinMax  Function=max  Inputs=2
  Relay : Relay  OnSwitchValue=hyst_min/2  OffSwitchValue=-hyst_min/2
  Sum : Sum  Inputs=-+|
  Switch1 : Switch  Criteria=u2 > Threshold
  Switch2 : Switch  Threshold=tmin*60
  Switch3 : Switch  Threshold=tmin*60
  Switch4 : Switch  Criteria=u2 > Threshold
  TVL-Regler nach t_a : MATLAB Function  TreatAsAtomicUnit=on
  St : Outport
  wires:
  Memory/1 -> Integrator/2
  Sum/1 -> Relay/1
  TVL-Regler nach t_a/1(TVL_SOLL) -> Sum/2
  Relay/1 -> Switch4/3, MinMax/1, MinMax1/1, Switch3/1
  Constant1/1 -> TVL-Regler nach t_a/3(TVLmin)
  Constant/1 -> TVL-Regler nach t_a/2(TVLmax)
  t_a/1 -> TVL-Regler nach t_a/1(t_a)
  t_IST/1 -> Sum/1
  Constant2/1 -> Switch1/1
  Constant3/1 -> Switch1/3
  Switch1/1 -> Integrator/1
  Switch2/1 -> Memory/1
  Constant4/1 -> Switch2/1
  Constant5/1 -> Switch2/3
  Integrator/1 -> Switch2/2, Switch4/2, Switch3/2
  Switch3/1 -> St/1, MinMax/2
  Switch4/1 -> Switch3/3
  MinMax/1 -> Switch1/2
  MinMax1/1 -> Switch4/1
  Constant7/1 -> MinMax1/2
  Constant6/1 -> TVL-Regler nach t_a/4(T_HG)

== system THAMO_6x2/Rohr ==
  note: Geodätische Höhe wird als const. Koeffizient aufaddiert
      |
      | Druckverlustberechnung im Rohr mittels Unterscheidung laminar/Übergangsbereich/Colebrook-White
  note: als klassische DGL für einen Knoten mit Wärmeverlust
  t___L : Inport
  THB__1_W : Inport  Port=2
  Bus Assignment : BusAssignment  AssignedSignals=Temperature,Pressure,DPConstant,DPLinear,DPQuadratic,GeodeticHeight
  Druckverlust : Subsystem  mask(theoretical pressure drop of a pipe){}
      mask help: Calculates the pressure drop in a pipe according to a theoretical model.
      mask Help: web(fullfile(path_carnot('help'),'Pressure_Drop_PipeTheory.html'),'-helpbrowser')
  Wärmeverlust : Subsystem  mask(theoretical pressure drop of a pipe){}
      mask help: Calculates the pressure drop in a pipe according to a theoretical model.
      mask Help: web(fullfile(path_carnot('help'),'Pressure_Drop_PipeTheory.html'),'-helpbrowser')
  THB : Outport
  wires:
  Druckverlust/5(Hgeo_2_W) -> Bus Assignment/7
  Druckverlust/4(dpq_2_W) -> Bus Assignment/6
  Druckverlust/3(dpl_2_W) -> Bus Assignment/5
  Druckverlust/2(dpc_2_W) -> Bus Assignment/4
  Wärmeverlust/1(t_2_W) -> Bus Assignment/2
  Bus Assignment/1 -> THB/1
  THB__1_W/1 -> Druckverlust/1(THB__1_W), Wärmeverlust/1(THB__1_W), Bus Assignment/1
  t___L/1 -> Wärmeverlust/2(t___L)
  Druckverlust/1(p_2_W) -> Bus Assignment/3

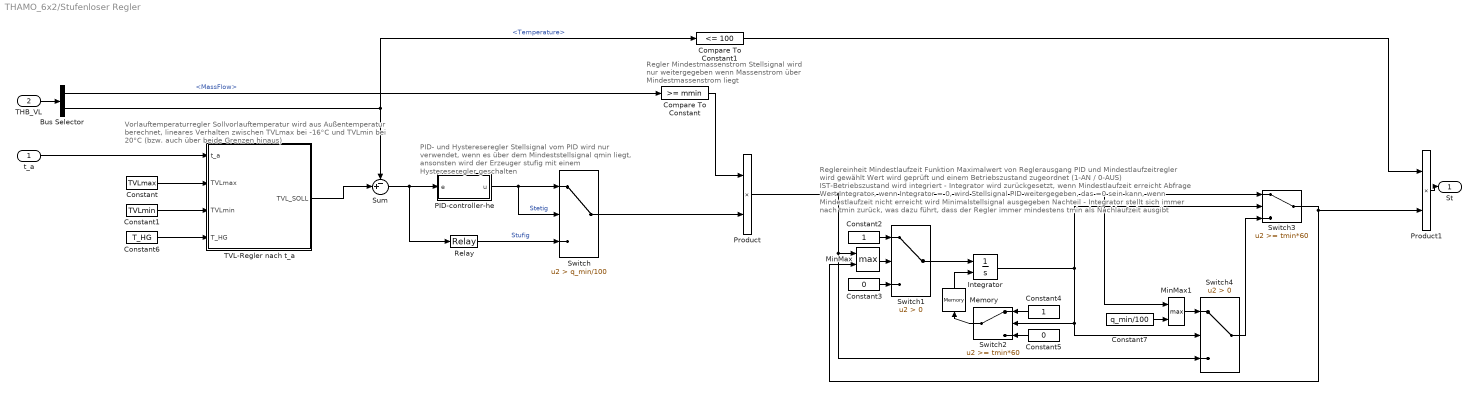
== system THAMO_6x2/Stufenloser Regler ==
  note: PID- und Hystereseregler
      |
      | Stellsignal vom PID wird nur verwendet, wenn es über dem Mindeststellsignal qmin liegt, ansonsten wird der
      | Erzeuger stufig mit einem Hystereseregler geschalten
  note: Vorlauftemperaturregler
      |
      | Sollvorlauftemperatur wird aus Außentemperatur berechnet, lineares Verhalten zwischen TVLmax bei -16°C und TVLmin bei 20°C (bzw. auch über beide Grenzen hinaus)
  note: Regler Mindestmassenstrom
      |
      | Stellsignal wird nur weitergegeben wenn Massenstrom über Mindestmassenstrom liegt
  note: Reglereinheit Mindestlaufzeit
      |
      | Funktion
      | Maximalwert von Reglerausgang PID und Mindestlaufzeitregler wird gewählt
      | Wert wird geprüft und einem Betriebszustand zugeordnet (1-AN / 0-AUS)
      | IST-Betriebszustand wird integriert - Integrator wird zurückgesetzt, wenn Mindestlaufzeit erreicht
      | Abfrage Wert Integrator, wenn Integrator = 0, wird Stellsignal PID weitergegeben, das =0 sein kann, wenn Mindestlaufzeit nicht erreicht wird Minimalstellsignal ausgegeben
      |
      | Nachteil
      | - Integrator stellt sich immer nach tmin zurück, was dazu führt, dass der Regler immer mindestens tmin als Nachlaufzeit ausgibt
  t_a : Inport
  THB_VL : Inport  Port=2
  Bus Selector : BusSelector  OutputSignals=MassFlow,Temperature
  Compare To Constant : simulink/Logic and Bit Operations/Compare To Constant  relop=>=  const=mmin  OutDataTypeStr=boolean
  Compare To Constant1 : simulink/Logic and Bit Operations/Compare To Constant  relop=<=  const=100  OutDataTypeStr=boolean
  Constant : Constant  Value=TVLmax
  Constant1 : Constant  Value=TVLmin
  Constant2 : Constant
  Constant3 : Constant  Value=0
  Constant4 : Constant
  Constant5 : Constant  Value=0
  Constant6 : Constant  Value=T_HG
  Constant7 : Constant  Value=q_min/100
  Integrator : Integrator  ExternalReset=level hold
  Memory : Memory  InitialCondition=1
  MinMax : MinMax  Function=max  Inputs=2
  MinMax1 : MinMax  Function=max  Inputs=2
  PID-controller-he : Subsystem  mask{Kp=Kp, Ki=Ki, Kd=Kd}
      mask prompts: Kp "Proportionalbeiwert Kp in 1/K"; Ki "Integralbeiwert Ki in 1/K*s"; Kd "Differentialbeiwert Kd in s/K"
  Product : Product
  Product1 : Product
  Relay : Relay  OnSwitchValue=hyst_min/2  OffSwitchValue=-hyst_min/2  OnOutputValue=q_min/100
  Sum : Sum  Inputs=-+|
  Switch : Switch  Criteria=u2 > Threshold  Threshold=q_min/100
  Switch1 : Switch  Criteria=u2 > Threshold
  Switch2 : Switch  Threshold=tmin*60
  Switch3 : Switch  Threshold=tmin*60
  Switch4 : Switch  Criteria=u2 > Threshold
  TVL-Regler nach t_a : MATLAB Function  TreatAsAtomicUnit=on
  St : Outport
  wires:
  Memory/1 -> Integrator/2
  PID-controller-he/1(u) -> Switch/1, Switch/2  "Stetig"
  Switch/1 -> Product/2
  Sum/1 -> Relay/1, PID-controller-he/1(e)
  TVL-Regler nach t_a/1(TVL_SOLL) -> Sum/2
  Relay/1 -> Switch/3  "Stufig"
  Compare To Constant/1 -> Product/1
  Bus Selector/1 -> Compare To Constant/1  "<MassFlow>"
  Product/1 -> MinMax1/1, Switch3/1, Switch4/3, MinMax/1
  Constant1/1 -> TVL-Regler nach t_a/3(TVLmin)
  Constant/1 -> TVL-Regler nach t_a/2(TVLmax)
  t_a/1 -> TVL-Regler nach t_a/1(t_a)
  Bus Selector/2 -> Sum/1, Compare To Constant1/1  "<Temperature>"
  THB_VL/1 -> Bus Selector/1
  Constant2/1 -> Switch1/1
  Constant3/1 -> Switch1/3
  Switch1/1 -> Integrator/1
  Switch2/1 -> Memory/1
  Constant4/1 -> Switch2/1
  Constant5/1 -> Switch2/3
  Integrator/1 -> Switch2/2, Switch4/2, Switch3/2
  Switch3/1 -> Product1/2, MinMax/2
  Switch4/1 -> Switch3/3
  MinMax/1 -> Switch1/2
  MinMax1/1 -> Switch4/1
  Constant7/1 -> MinMax1/2
  Constant6/1 -> TVL-Regler nach t_a/4(T_HG)
  Compare To Constant1/1 -> Product1/1
  Product1/1 -> St/1

== system THAMO_6x2/T-Stueck mischend ==
  THB1 : Inport
  THB2 : Inport  Port=2
  clq : Inport  Port=3
  Mixer : Subsystem
  PT1_for_fdiv : Subsystem
  THB : Outport
  fdiv : Outport  Port=2
  wires:
  Mixer/2(ID1) -> PT1_for_fdiv/1(ID_1)
  Mixer/3(ID2) -> PT1_for_fdiv/2(ID_2)
  Mixer/4(fdiv) -> PT1_for_fdiv/3(fdiv)
  THB2/1 -> Mixer/3(THB2)
  Mixer/1(THB) -> THB/1
  THB1/1 -> Mixer/1(THB1)
  PT1_for_fdiv/1(f_div) -> fdiv/1
  clq/1 -> Mixer/2(clq)

== system THAMO_6x2/T-Stueck trennend ==
  THB : Inport
  fdiv : Inport  Port=2
  Bus Assignment : BusAssignment  AssignedSignals=ID,MassFlow,DPConstant,DPLinear,DPQuadratic
  Bus Assignment1 : BusAssignment  AssignedSignals=ID,MassFlow,DPConstant,DPLinear,DPQuadratic
  Bus Selector : BusSelector  OutputSignals=MassFlow
  Bus Selector4 : BusSelector  OutputSignals=ID
  Dot Product : DotProduct  InputSameDT=on  OutDataTypeStr=Inherit: Inherit via internal rule
  Saturation : Saturate  UpperLimit=1  LowerLimit=0
  Sum : Sum  Inputs=-+  SaturateOnIntegerOverflow=on  InputSameDT=on  OutDataTypeStr=Inherit: Same as first input
  const{,1..2,4..6} (6 alike) : Constant  Value=0
  increase_ID : Subsystem
  THB1 : Outport
  THB2 : Outport  Port=2
  clq : Outport  Port=3
  wires:
  const2/1 -> Bus Assignment1/6  "DPQuadratic"
  const1/1 -> Bus Assignment1/5  "DPLinear"
  Saturation/1 -> Dot Product/2
  Sum/1 -> Bus Assignment1/3  "MassFlow"
  Bus Selector/1 -> Dot Product/1, Sum/2  "<MassFlow>"
  const/1 -> Bus Assignment1/4  "DPConstant"
  fdiv/1 -> Saturation/1
  Dot Product/1 -> Sum/1, Bus Assignment/3  "MassFlow"
  Bus Selector4/1 -> increase_ID/1(In1)  "<ID>"
  increase_ID/1(Out1) -> Bus Assignment/2, Bus Assignment1/2  "ID"
  const6/1 -> Bus Assignment/6  "DPQuadratic"
  const5/1 -> Bus Assignment/5  "DPLinear"
  const4/1 -> Bus Assignment/4  "DPConstant"
  Bus Assignment/1 -> THB1/1
  Bus Assignment1/1 -> THB2/1
  THB/1 -> clq/1, Bus Selector/1, Bus Assignment/1, Bus Selector4/1, Bus Assignment1/1
